simulink model "remake"  (R2026a)
settings: Solver=FixedStepAuto  StopTime=50  FixedStep=0.001
values from neighbouring files (symbols this model uses):
  brake_bias_f = 0.60    (= 0.6)    [setupParams.m]    (also in setupParamsSingle.m)
  brake_bias_r = 1 - brake_bias_f    (= 0.4)    [setupParams.m]    (also in setupParamsSingle.m)
  camber_front = -1.5    [setupParams.m]    (also in setupParamsSingle.m)
  camber_rear = -1    [setupParams.m]    (also in setupParamsSingle.m)
  gnd_displ = 0.0    (= 0)    [setupParams.m]    (also in setupParamsSingle.m)
  l_f = 0.775    [setupParams.m]    (also in setupParamsSingle.m)
  l_r = 0.775    [setupParams.m]    (also in setupParamsSingle.m)
  pa_front_wheel = 82700    [setupParams.m]    (also in setupParamsSingle.m)
  pa_rear_wheel = 82700    [setupParams.m]    (also in setupParamsSingle.m)
  scale_factor_front = ones(27, 1)    [setupParams.m]    (also in setupParamsSingle.m)
  scale_factor_rear = ones(27, 1)    [setupParams.m]    (also in setupParamsSingle.m)
  track_width_f = 1.2    [setupParams.m]    (also in setupParamsSingle.m)
  track_width_r = 1.2    [setupParams.m]    (also in setupParamsSingle.m)
  Ts = 0.01    [setupParams.m]    (also in setupParamsSingle.m)
libraries: simulink x30, vehdynlibtire x4, sim3dlib x1, vehdynlibsteering x1, autolibshared x1, sim3dautolib x1
(part 1 of 3)
settings Model: SimulationMode=accelerator  Creator=Utente  LastModifiedBy=Utente
settings SolverCC: ZeroCrossControl=DisableAll  EnableFixedStepZeroCrossing=on

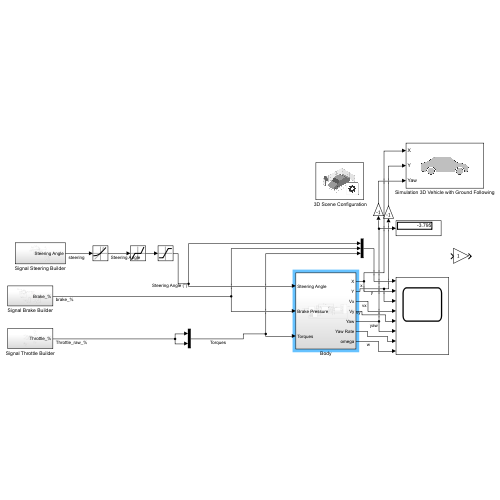
[thumbnail: Simulink's stored preview of the top-level diagram]
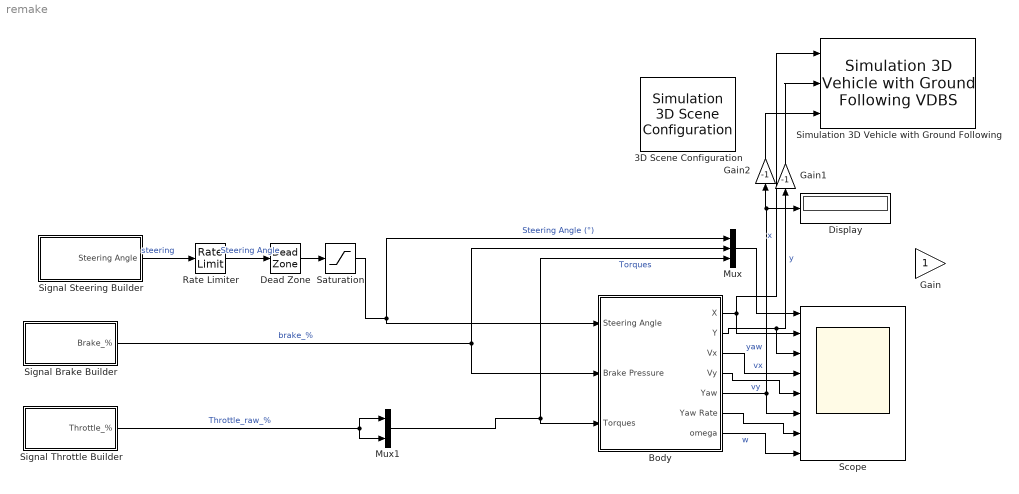
== system remake ==
  " 3D Scene Configuration" : sim3dlib/Simulation 3D Scene Configuration  Priority=0  ProjectFormat=Default Scenes  SceneDesc=Open surface  ProjectName=Z:\.Programmi\MATLAB26a\toolbox\shared\sim3d_projects\automotive_project_windows\UE\WindowsNoEditor\VehicleSimulation.exe  ScenePath=/Game/Maps/HwStrght  EnableOpenDRIVE=off  vehTagList={'Custom';'Scene Origin';'SimulinkVehicle1'}  vehTag=SimulinkVehicle1  AttachedCameraRelativeTranslation=[0 0 0]  FreeCameraDefaultInitialTranslation=[-6, 0, 2]  AttachedCameraRelativeRotation=[0 0 0]  FreeCameraDefaultInitialRotation=[0, -15, 0]  ViewpointName=Custom  FreeCameraInitialTranslation=[0 0 0]  FreeCameraInitialRotation=[0 0 0]  OpVisEn=off  Ts=.03  EnableWindow=on  EnableRemoteAccess=off  SimulationMode=CoSimulation  SimulateUsing=Interpreted execution  EnableAnimationRecording=off  OverrideDefaultRecording=off  AnimationRecordingFileName=sim3dAnimation.mat  AnimationRecordingInterval=[0 inf]  EnableWeather=off  SunAzimuth=90  SunAltitude=40.0  EnableGeospatialSun=off  Latitude=0  Longitude=0  Date=2023-01-01  Time=10:30:00  GeoTimeZone=-5.0  SunDaylightSaving=off  wind=1  clouds=10  EnableVolumetricClouds=off  CloudCoverage=0  CloudAltitude=6  fog=0  rain=0  RaindropsEffect=off  SnowDensity=0  EnableGeospatial=off  TilesetSource=Earth terrain  UseTrueOrigin=off  OriginHeight=200  OriginLatitude=40.744652  OriginLongitude=-73.988864  MapStyle=Aerial  AdditionalAssetIDs=[]  UseAdvancedSunSky=off  SolarTime=11  TimeZone=-5  Day=21  Month=9  Year=2022  UseDaylightSavingTime=on  DSTStartDay=10  DSTStartMonth=3  DSTEndDay=3  DSTEndMonth=11  DSTSwitchHour=2  sensorTag=MainCamera1  sensorId=1  sensorName=MainCamera1  mountLoc=Origin  offsetFlag=off  tmountOffset=[0, 0, 0]  rmountOffset=[0, 0, 0]  HorizontalResolution=1280  VerticalResolution=720  HorizontalFOV=60  mountPoint=[0 0 0]  mountOrientation=[0 0 0]  aMode=2  ID=1  GeoTrigger=Inactive  ViewNameList={'Custom'}  ViewTranslationList={'[0 0 0]'}  ViewRotationList={'[0 0 0]'}
      settings: LibrarySourceBlock=vehdynlibsim3dcore/Simulation 3D Scene Configuration
  Body : Subsystem
  Dead Zone : DeadZone  LowerValue=-2  UpperValue=2
  Display : Display
  Gain : Gain
  Gain1 : Gain  Gain=-1
  Gain2 : Gain  Gain=-1
  Mux : Mux  Inputs=3
  Mux1 : Mux  Inputs=2
  Rate Limiter : RateLimiter  RisingSlewLimit=150  FallingSlewLimit=-150  SampleTimeMode=inherited
  Saturation : Saturate  UpperLimit=130  LowerLimit=-130
  Scope : Scope  NumInputPorts=8
      settings: ActiveDisplayYMinimum=-72.499999999999986  ActiveDisplayYMaximum=72.499999999999929
  Signal Brake Builder : Subsystem
  Signal Steering Builder : Subsystem
  Signal Throttle Builder : Subsystem
  Simulation 3D Vehicle with Ground Following : sim3dautolib/Simulation 3D Vehicle with Ground Following VDBS  Priority=-1  PassVehMesh=Formula student vehicle  MeshPath=/MathWorksAutomotiveContent/Vehicles/Muscle/Meshes/SK_MuscleCar.SK_MuscleCar  TrackWidth=1.9  WheelBase=3  WheelRadius=0.35  VehColor=Red  CoordinateSystem=SAE  InitialPos=[0, 0, 0]  InitialRot=[0,0,0]  ActorName=SimulinkVehicle1  VehLightsControl=off  HeadlightColor=[ 1, 1, 1 ]  HighBeamIntensity=100000  LowBeamIntensity=60000  HighBeamConeAngle=1.22  LowBeamConeAngle=1.22  LeftHeadlightOrientation=[ 0, 0 ]  RightHeadlightOrientation=[ 0, 0 ]  BrakelightIntensity=200  ReverselightIntensity=500  SignallightIntensity=500  SignallightPeriod=1  SignalPulseWidth=50  SampleTime=-1  ActorType=SimulinkVehicle  ID=1  aMode=2  ActorTag=SimulinkVehicle1  CoordinateScheme=0
      settings: LibrarySourceBlock=vehdynlibsim3d/Simulation 3D Vehicle with Ground Following
  wires:
  Signal Steering Builder/1(Steering Angle) -> Rate Limiter/1  "steering"
  Signal Brake Builder/1(Brake_%) -> Mux/2, Body/2(Brake Pressure)  "brake_%"
  Body/1(X) -> Simulation 3D Vehicle with Ground Following/1, Scope/2  "x"
  Body/2(Y) -> Gain1/1, Scope/3  "y"
  Body/3(Vx) -> Scope/4  "vx"
  Body/4(Vy) -> Scope/5  "vy"
  Body/5(Yaw) -> Scope/6, Display/1, Gain2/1  "yaw"
  Body/7(omega) -> Scope/8  "w"
  Mux/1 -> Scope/1
  Signal Throttle Builder/1(Throttle_%) -> Mux1/1, Mux1/2  "Throttle_raw_%"
  Mux1/1 -> Mux/3, Body/3(Torques)  "Torques"
  Rate Limiter/1 -> Dead Zone/1  "Steering Angle"
  Dead Zone/1 -> Saturation/1
  Saturation/1 -> Mux/1, Body/1(Steering Angle)  "Steering Angle (°)"
  Body/6(Yaw Rate) -> Scope/7
  Gain1/1 -> Simulation 3D Vehicle with Ground Following/2
  Gain2/1 -> Simulation 3D Vehicle with Ground Following/3

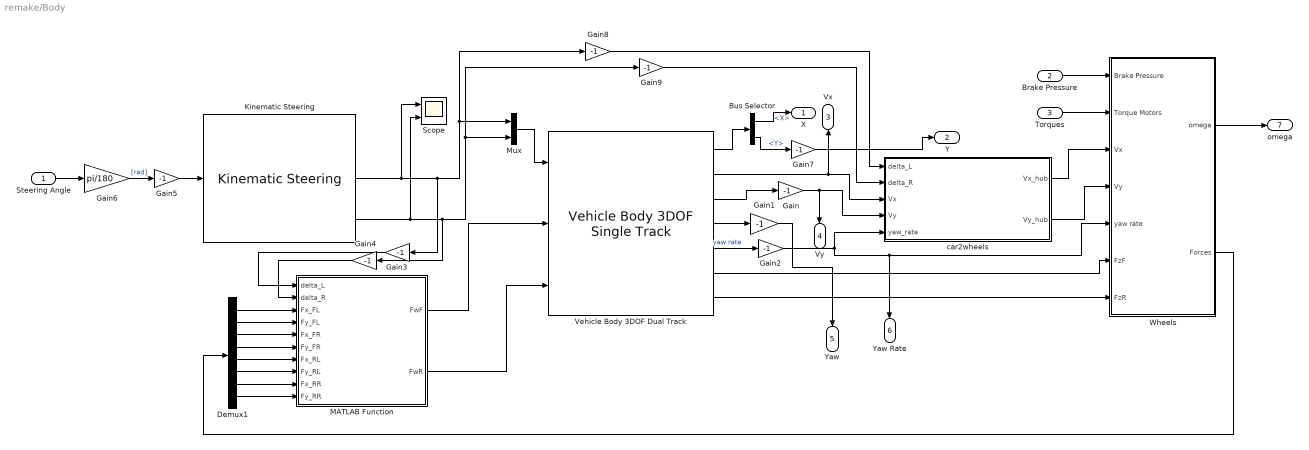
== system remake/Body ==
  Steering Angle : Inport
  Brake Pressure : Inport  Port=2
  Torques : Inport  Port=3
  Bus Selector : BusSelector  OutputSignals=InertFrm.Cg.Disp.X,InertFrm.Cg.Disp.Y
  Demux1 : Demux  Outputs=8
  Gain{,1..5,7..9} (9 alike) : Gain  Gain=-1
  Gain6 : Gain  Gain=pi/180
  Kinematic Steering : vehdynlibsteering/Kinematic Steering  StrgType=Ackerman  StrgRatioType=Constant  Loc=Front  NrmlFctr=0.01  TrckWdth=1.2  WhlBase=1.55  Db=0  StrgRng=pi  StrgAngBpts="[-6.2832   -5.0265   -3.7699   -2.5133   -1.2566         0    1.2566    2.5133    3.7699    5.0265    6.2832]"  StrgRatioTbl=|  StrgRatio=4.2  PctAckIn=off  PctAck=100  PctAckTbl=ones(1,11)*100  StrgArmLngth=0.1  RckCsLngth=0.5  TieRodLngth=0.248  D=0.2  PnnRadius=0.00085818  PnnRadiusTbl="[0.0055    0.0055    0.0056    0.0057    0.0058    0.0057    0.0057    0.0057    0.0056    0.0055    0.0055]"  RodLngth=0.1  ParaArmLngth=0.9  aMode=2
      | [13.5000   13.3750   13.2500   13.1250   13.0000   13.0000   13.0000   13.1250   13.2500   13.3750   13.5000
      | ]
  MATLAB Function : MATLAB Function  TreatAsAtomicUnit=on
  Mux : Mux  Inputs=2
  Scope : Scope  NumInputPorts=2
      settings: ActiveDisplayYMinimum=-0.19369023585862366  ActiveDisplayYMaximum=0.062259490327338275
  Vehicle Body 3DOF Dual Track : autolibshared/Vehicle Body 3DOF Single Track  trackMode=Dual  inputMode=External forces  frontSteerMode=on  rearSteerMode=off  extFMode=off  htchFMode=off  extMMode=off  htchMMode=off  windMode=off  extTamb=off  muMode=off  extGndPlnElev=off  extGndPlnRoll=off  extGndPlnPitch=off  extGndPlnDCM=off  extXo=off  extxdoto=off  extYo=off  extydoto=off  extpsio=off  extro=off  aMode=2  NF=2  NR=2  m=320  a=0.775  b=0.775  h=0.35  dh=1  hh=0.2  X_o=0  xdot_o=0  d=0  hl=0  w=[1.2,1.2]  CalphaMode=Constant  sigmaMode=on  sigma_f=.1  sigma_r=.1  Cy_f=12e3  Cy_r=11e3  Cy_f_data="[1.396121365092108e+04\t4.232462640127975e+04\t6.754894575573687e+04\t8.835784428391886e+04\t1.043551700699839e+05\t1.158335754468729e+05\t1.234691551560788e+05\t1.280575366661118e+05\t1.298126639907242e+05\t1.298126639907242e+05]"  alpha_f_brk=[-0.785, -0.628, -0.471, -0.314, -0.157, 0.000, 0.157, 0.314, 0.471, 0.628, 0.785]  Fz_f_brk="[500\t1.555555555555556e+03\t2.611111111111111e+03\t3.666666666666667e+03\t4.722222222222223e+03\t5.777777777777777e+03\t6.833333333333333e+03\t7.888888888888889e+03\t8.944444444444445e+03\t10000]"  Cy_r_data="[1.396121365092108e+04\t4.232462640127975e+04\t6.754894575573687e+04\t8.835784428391886e+04\t1.043551700699839e+05\t1.158335754468729e+05\t1.234691551560788e+05\t1.280575366661118e+05\t1.298126639907242e+05\t1.298126639907242e+05]"  alpha_r_brk=[-0.785, -0.628, -0.471, -0.314, -0.157, 0.000, 0.157, 0.314, 0.471, 0.628, 0.785]  Fz_r_brk="[500\t1.555555555555556e+03\t2.611111111111111e+03\t3.666666666666667e+03\t4.722222222222223e+03\t5.777777777777777e+03\t6.833333333333333e+03\t7.888888888888889e+03\t8.944444444444445e+03\t10000]"  Fznom=5000  Y_o=0  ydot_o=0  Izz=200  psi_o=0  r_o=0  Af=1.1  Cd=1.3  Cl=1  Cpm=.1  beta_w=[0 0.01:0.01:0.3]  Cs=[0:0.03:0.9]  Cym=[0 1e-6:0.01:0.3]  Pabs=101325  Tair=273  g=9.81  mu=1  GndPlnRoll=0  GndPlnPitch=0  GndPlnElev=0  xdot_tol=.01  Fxtire_sat=7e4  Fytire_sat=7e4  longOff=0  latOff=0  vertOff=0  wrapAng=off
      settings: LibrarySourceBlock=vehdynlibeom/Vehicle Body 3DOF Dual Track
  Wheels : Subsystem
  car2wheels : MATLAB Function  TreatAsAtomicUnit=on
  X : Outport
  Y : Outport  Port=2
  Vx : Outport  Port=3
  Vy : Outport  Port=4
  Yaw : Outport  Port=5
  Yaw Rate : Outport  Port=6
  omega : Outport  Port=7
  wires:
  Gain/1 -> car2wheels/4(Vy), Vy/1
  Demux1/2 -> MATLAB Function/4(Fy_FL)
  Vehicle Body 3DOF Dual Track/1 -> Bus Selector/1
  Vehicle Body 3DOF Dual Track/4 -> Gain1/1
  Gain2/1 -> car2wheels/5(yaw_rate), Yaw Rate/1, Wheels/5(yaw rate)
  Demux1/5 -> MATLAB Function/7(Fx_RL)
  Vehicle Body 3DOF Dual Track/3 -> Gain/1
  Vehicle Body 3DOF Dual Track/2 -> Vx/1, car2wheels/3(Vx)
  Wheels/1(omega) -> omega/1
  Vehicle Body 3DOF Dual Track/6 -> Wheels/6(FzF)
  Demux1/7 -> MATLAB Function/9(Fx_RR)
  Demux1/8 -> MATLAB Function/10(Fy_RR)
  Vehicle Body 3DOF Dual Track/5 -> Gain2/1  "yaw rate"
  Demux1/6 -> MATLAB Function/8(Fy_RL)
  Demux1/4 -> MATLAB Function/6(Fy_FR)
  MATLAB Function/1(FwF) -> Vehicle Body 3DOF Dual Track/2
  Demux1/3 -> MATLAB Function/5(Fx_FR)
  car2wheels/2(Vy_hub) -> Wheels/4(Vy)
  Demux1/1 -> MATLAB Function/3(Fx_FL)
  Bus Selector/2 -> Gain7/1  "<Y>"
  Torques/1 -> Wheels/2(Torque Motors)
  Steering Angle/1 -> Gain6/1
  Vehicle Body 3DOF Dual Track/7 -> Wheels/7(FzR)
  Bus Selector/1 -> X/1  "<X>"
  Wheels/2(Forces) -> Demux1/1
  MATLAB Function/2(FwR) -> Vehicle Body 3DOF Dual Track/3
  Gain5/1 -> Kinematic Steering/1
  Mux/1 -> Vehicle Body 3DOF Dual Track/1
  Brake Pressure/1 -> Wheels/1(Brake Pressure)
  Gain6/1 -> Gain5/1  "[rad]"
  car2wheels/1(Vx_hub) -> Wheels/3(Vx)
  Gain1/1 -> Yaw/1
  Kinematic Steering/2 -> Scope/1, Gain3/1, Gain8/1, Mux/1
  Kinematic Steering/3 -> Scope/2, Gain4/1, Gain9/1, Mux/2
  Gain3/1 -> MATLAB Function/1(delta_L)
  Gain4/1 -> MATLAB Function/2(delta_R)
  Gain8/1 -> car2wheels/1(delta_L)
  Gain9/1 -> car2wheels/2(delta_R)
  Gain7/1 -> Y/1

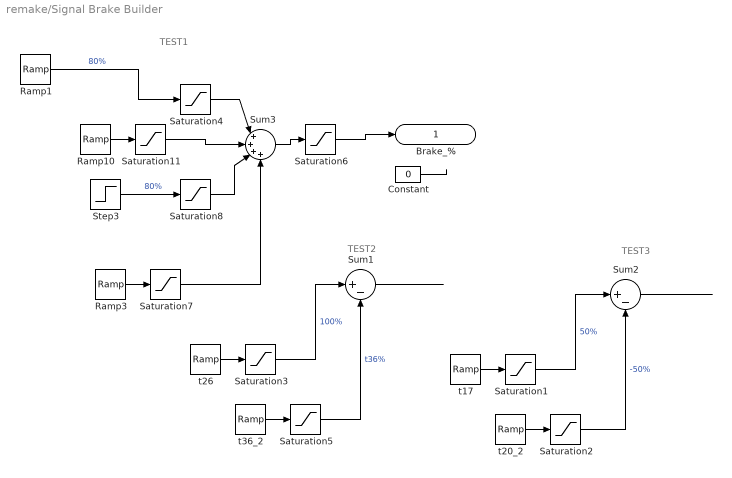
== system remake/Signal Brake Builder ==
  note: TEST2
  note: TEST1
  note: TEST3
  Constant : Constant  Value=0
  Ramp1 : simulink/Sources/Ramp  slope=50  start=20  InitialOutput=0
  Ramp10 : simulink/Sources/Ramp  slope=-30  start=21  InitialOutput=0
  Ramp3 : simulink/Sources/Ramp  slope=-30  start=33.5  InitialOutput=0
  Saturation1 : Saturate  UpperLimit=50  LowerLimit=-70
  Saturation{3,5,7,11} (4 alike) : Saturate  UpperLimit=100  LowerLimit=-70
  Saturation2 : Saturate  UpperLimit=50  LowerLimit=-50
  Saturation4 : Saturate  UpperLimit=70  LowerLimit=0
  Saturation6 : Saturate  UpperLimit=100  LowerLimit=0
  Saturation8 : Saturate  UpperLimit=70  LowerLimit=0
  Step3 : Step  Time=33  FinalValue=30  SampleTime=0
  Sum1 : Sum  Inputs=|+-
  Sum2 : Sum  Inputs=|+-
  Sum3 : Sum  Inputs=|++++
  t17 : simulink/Sources/Ramp  slope=50  start=17  InitialOutput=0
  t20_2 : simulink/Sources/Ramp  slope=+50  start=20  InitialOutput=0
  t26 : simulink/Sources/Ramp  slope=50  start=26  InitialOutput=0
  t36_2 : simulink/Sources/Ramp  slope=50  start=36  InitialOutput=0
  Brake_% : Outport
  wires:
  Constant/1 -> ?
  Sum1/1 -> ?
  t17/1 -> Saturation1/1
  Saturation4/1 -> Sum3/1
  Saturation1/1 -> Sum2/1  "50%"
  Sum3/1 -> Saturation6/1
  Saturation8/1 -> Sum3/3
  Saturation6/1 -> Brake_%/1
  Ramp3/1 -> Saturation7/1
  Sum2/1 -> ?
  t26/1 -> Saturation3/1
  Saturation2/1 -> Sum2/2  "-50%"
  Saturation7/1 -> Sum3/4
  Ramp1/1 -> Saturation4/1  "80%"
  Saturation3/1 -> Sum1/1  "100%"
  t36_2/1 -> Saturation5/1
  Ramp10/1 -> Saturation11/1
  t20_2/1 -> Saturation2/1
  Saturation5/1 -> Sum1/2  "t36%"
  Saturation11/1 -> Sum3/2
  Step3/1 -> Saturation8/1  "80%"

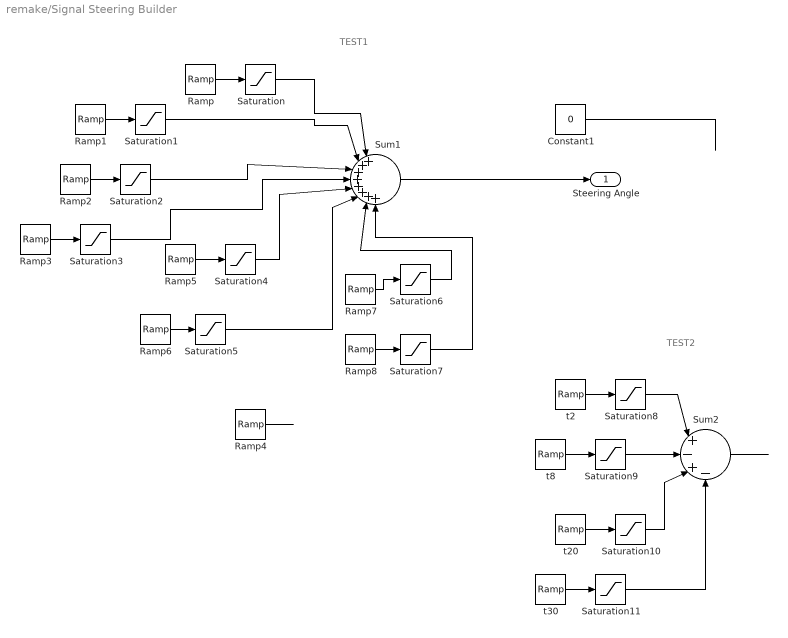
== system remake/Signal Steering Builder ==
  note: TEST2
  note: TEST1
  Constant1 : Constant  Value=0
  Ramp : simulink/Sources/Ramp  slope=20  start=3  InitialOutput=0
  Ramp1 : simulink/Sources/Ramp  slope=-20  start=7  InitialOutput=0
  Ramp2 : simulink/Sources/Ramp  slope=-30  start=7  InitialOutput=0
  Ramp3 : simulink/Sources/Ramp  slope=20  start=11  InitialOutput=0
  Ramp4 : simulink/Sources/Ramp  slope=30  start=4  InitialOutput=0
  Ramp5 : simulink/Sources/Ramp  slope=30  start=25  InitialOutput=0
  Ramp6 : simulink/Sources/Ramp  slope=-20  start=27  InitialOutput=0
  Ramp7 : simulink/Sources/Ramp  slope=-40  start=35  InitialOutput=0
  Ramp8 : simulink/Sources/Ramp  slope=30  start=37  InitialOutput=0
  Saturation{,1..5} (6 alike) : Saturate  UpperLimit=40  LowerLimit=-40
  Saturation{8..11} (4 alike) : Saturate  UpperLimit=50  LowerLimit=-50
  Saturation6 : Saturate  UpperLimit=60  LowerLimit=-60
  Saturation7 : Saturate  UpperLimit=60  LowerLimit=-60
  Sum1 : Sum  Inputs=|++++++++
  Sum2 : Sum  Inputs=|+-+-
  t2 : simulink/Sources/Ramp  slope=20  start=2  InitialOutput=0
  t20 : simulink/Sources/Ramp  slope=-20  start=20  InitialOutput=0
  t30 : simulink/Sources/Ramp  slope=-20  start=30  InitialOutput=0
  t8 : simulink/Sources/Ramp  slope=20  start=8  InitialOutput=0
  Steering Angle : Outport
  wires:
  Ramp4/1 -> ?
  Constant1/1 -> ?
  Sum2/1 -> ?
  Saturation9/1 -> Sum2/2
  t30/1 -> Saturation11/1
  Ramp1/1 -> Saturation1/1
  Ramp7/1 -> Saturation6/1
  Saturation2/1 -> Sum1/3
  Saturation10/1 -> Sum2/3
  Saturation3/1 -> Sum1/4
  Ramp3/1 -> Saturation3/1
  Saturation11/1 -> Sum2/4
  Saturation7/1 -> Sum1/8
  Saturation/1 -> Sum1/1
  t2/1 -> Saturation8/1
  t20/1 -> Saturation10/1
  Ramp8/1 -> Saturation7/1
  Ramp5/1 -> Saturation4/1
  Saturation8/1 -> Sum2/1
  Saturation1/1 -> Sum1/2
  Ramp2/1 -> Saturation2/1
  t8/1 -> Saturation9/1
  Sum1/1 -> Steering Angle/1
  Saturation5/1 -> Sum1/6
  Saturation6/1 -> Sum1/7
  Ramp/1 -> Saturation/1
  Saturation4/1 -> Sum1/5
  Ramp6/1 -> Saturation5/1

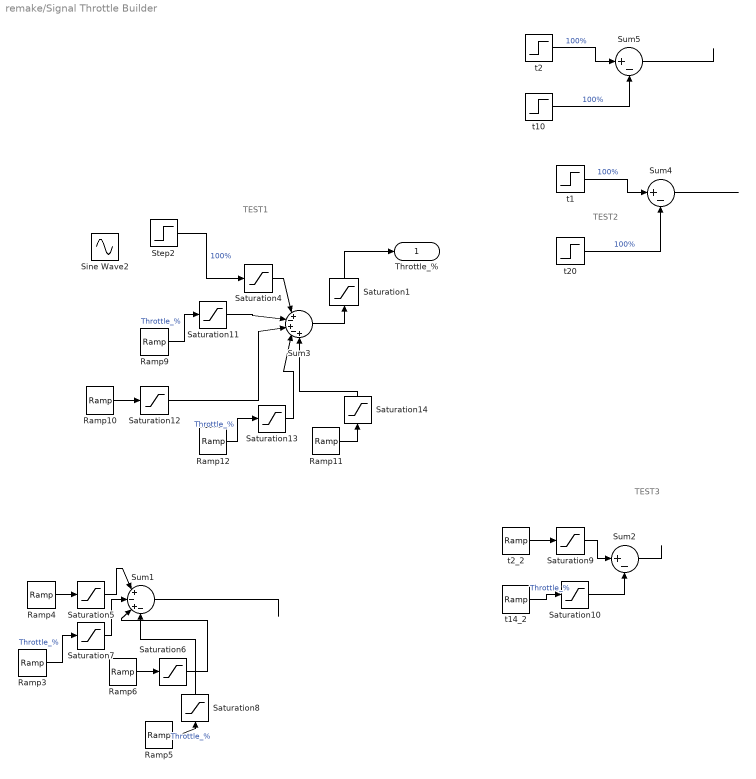
== system remake/Signal Throttle Builder ==
  note: TEST1
  note: TEST2
  note: TEST3
  Ramp10 : simulink/Sources/Ramp  slope=50  start=26  InitialOutput=0
  Ramp11 : simulink/Sources/Ramp  slope=12  start=34  InitialOutput=0
  Ramp12 : simulink/Sources/Ramp  slope=100  start=31  InitialOutput=0
  Ramp3 : simulink/Sources/Ramp  slope=50  start=8  InitialOutput=0
  Ramp4 : simulink/Sources/Ramp  slope=150  start=1  InitialOutput=0
  Ramp5 : simulink/Sources/Ramp  slope=100  start=20  InitialOutput=0
  Ramp6 : simulink/Sources/Ramp  slope=50  start=12  InitialOutput=0
  Ramp9 : simulink/Sources/Ramp  slope=100  start=19  InitialOutput=0
  Saturation1 : Saturate  UpperLimit=50  LowerLimit=0
  Saturation{4..14} (11 alike) : Saturate  UpperLimit=100  LowerLimit=0
  Sine Wave2 : Sin  Amplitude=800  Frequency=0.3  SampleTime=Ts
  Step2 : Step  Time=2  FinalValue=100  SampleTime=0
  Sum1 : Sum  Inputs=|+-+-
  Sum2 : Sum  Inputs=|+-
  Sum3 : Sum  Inputs=|+-+-+
  Sum4 : Sum  Inputs=|+-
  Sum5 : Sum  Inputs=|+-
  t1 : Step  FinalValue=100  SampleTime=0
  t10 : Step  Time=10  FinalValue=100  SampleTime=0
  t14_2 : simulink/Sources/Ramp  slope=50  start=14  InitialOutput=0
  t2 : Step  FinalValue=100  SampleTime=0
  t20 : Step  Time=20  FinalValue=100  SampleTime=0
  t2_2 : simulink/Sources/Ramp  slope=50  start=2  InitialOutput=0
  Throttle_% : Outport
  wires:
  Sum4/1 -> ?
  Sum1/1 -> ?
  Sum2/1 -> ?
  Sum5/1 -> ?
  Step2/1 -> Saturation4/1  "100%"
  Ramp10/1 -> Saturation12/1
  Saturation7/1 -> Sum1/2
  Saturation13/1 -> Sum3/4
  Ramp9/1 -> Saturation11/1  "Throttle_%"
  t10/1 -> Sum5/2  "100%"
  Saturation5/1 -> Sum1/1
  Ramp6/1 -> Saturation6/1
  Saturation9/1 -> Sum2/1
  t2_2/1 -> Saturation9/1
  Saturation14/1 -> Sum3/5
  Saturation10/1 -> Sum2/2
  Saturation8/1 -> Sum1/4
  Saturation6/1 -> Sum1/3
  t1/1 -> Sum4/1  "100%"
  Ramp5/1 -> Saturation8/1  "Throttle_%"
  Sum3/1 -> Saturation1/1
  Ramp3/1 -> Saturation7/1  "Throttle_%"
  t20/1 -> Sum4/2  "100%"
  t2/1 -> Sum5/1  "100%"
  Ramp4/1 -> Saturation5/1
  Saturation11/1 -> Sum3/2
  Ramp12/1 -> Saturation13/1  "Throttle_%"
  Ramp11/1 -> Saturation14/1
  t14_2/1 -> Saturation10/1  "Throttle_%"
  Saturation12/1 -> Sum3/3
  Saturation4/1 -> Sum3/1
  Saturation1/1 -> Throttle_%/1
